simulink model "FRNmodel_IMHRC"  (Simulink 7.9)
settings: Solver=VariableStepDiscrete  StartTime=0.0  StopTime=100.0  RelTol=1e-3
libraries: simeventslib x30
(part 2 of 3)

== system FRNmodel_IMHRC/FastCartonSTORE/Calculate_INFlow ==
  Calculate_INFlow : MATLAB Function  TreatAsAtomicUnit=on
  Entity Combiner : EntityCombiner  NumberInputPorts=2
  Entity Sink : EntitySink
  Entity Splitter : EntitySplitter  NumberOutputPorts=2
  FIFO Queue : FIFOQueue  Capacity=inf
  Get Attribute : GetAttribute  AttributeName=UoH|Quantity|INFlow  AttributeMissing=Error|Error|Error  AttributeDefaultValue=1|1|1  AttributeTreatAsVector=1|1|1  AttributeSendTiming=After entity departure|After entity departure|After entity departure  EvaluatedDefaultAttributeValue={[];[];[]}
      settings: OutputPortMap=o1,o2,o3
  Set Attribute : SetAttribute  AttributeName=INFlow  AttributeFrom=Signal port  EvaluatedAttributeValue={[]}
  Single Server : SingleServer  ServiceTime=0
  FlowRecord_IN : PMIOPort  Port=1  Side=Right
  FlowRecord_OUT : PMIOPort  Port=2  Side=Right
  INFlow_Signal : PMIOPort  Port=3  Side=Left
  wires:
  Get Attribute/1 -> Calculate_INFlow/1(UoH)
  Calculate_INFlow/1(INFlow_return) -> Set Attribute/1
  Get Attribute/2 -> Calculate_INFlow/2(Quantity)
  Get Attribute/3 -> Calculate_INFlow/3(INFlow)
  connections:
  Entity Combiner/RConn1 -- Get Attribute/LConn1
  Set Attribute/RConn1 -- Entity Splitter/LConn1
  Get Attribute/RConn1 -- Single Server/LConn1
  Single Server/RConn1 -- Set Attribute/LConn1
  FlowRecord_OUT/RConn1 -- Entity Splitter/RConn1
  FlowRecord_IN/RConn1 -- Entity Combiner/LConn1
  Entity Splitter/RConn2 -- Entity Sink/LConn1
  INFlow_Signal/RConn1 -- FIFO Queue/LConn1
  FIFO Queue/RConn1 -- Entity Combiner/LConn2

== system FRNmodel_IMHRC/FastCartonSTORE/Calculate_OUTFlow ==
  Calculate_OUTFlow : MATLAB Function  TreatAsAtomicUnit=on
  Entity Combiner : EntityCombiner  NumberInputPorts=2
  Entity Sink : EntitySink
  Entity Splitter : EntitySplitter  NumberOutputPorts=2
  FIFO Queue : FIFOQueue  Capacity=inf
  Get Attribute : GetAttribute  AttributeName=UoH|Quantity|OUTFlow  AttributeMissing=Error|Error|Error  AttributeDefaultValue=1|1|1  AttributeTreatAsVector=1|1|1  AttributeSendTiming=After entity departure|After entity departure|After entity departure  EvaluatedDefaultAttributeValue={[];[];[]}
      settings: OutputPortMap=o1,o2,o3
  Set Attribute : SetAttribute  AttributeName=OUTFlow  AttributeFrom=Signal port  EvaluatedAttributeValue={[]}
  Single Server : SingleServer  ServiceTime=0
  FlowRecord_IN : PMIOPort  Port=1  Side=Left
  FlowRecord_OUT : PMIOPort  Port=2  Side=Left
  OUTFlow_Signal : PMIOPort  Port=3  Side=Right
  wires:
  Get Attribute/1 -> Calculate_OUTFlow/1(UoH)
  Calculate_OUTFlow/1(OUTFlow_return) -> Set Attribute/1
  Get Attribute/2 -> Calculate_OUTFlow/2(Quantity)
  Get Attribute/3 -> Calculate_OUTFlow/3(OUTFlow)
  connections:
  Entity Combiner/RConn1 -- Get Attribute/LConn1
  Set Attribute/RConn1 -- Entity Splitter/LConn1
  Get Attribute/RConn1 -- Single Server/LConn1
  Single Server/RConn1 -- Set Attribute/LConn1
  FlowRecord_OUT/RConn1 -- Entity Splitter/RConn1
  FlowRecord_IN/RConn1 -- Entity Combiner/LConn1
  OUTFlow_Signal/RConn1 -- FIFO Queue/LConn1
  FIFO Queue/RConn1 -- Entity Combiner/LConn2
  Entity Splitter/RConn2 -- Entity Sink/LConn1

== system FRNmodel_IMHRC/FastCartonSTORE/FRN_Process ==
  FIFO Queue1 : FIFOQueue
  N-Server : NServer  NumberOfServers=inf  ServiceTime=0
  Flow_IN : PMIOPort  Port=1  Side=Left
  Message_IN : PMIOPort  Port=2  Side=Left
  Flow_OUT : PMIOPort  Port=3  Side=Right
  Message_OUT : PMIOPort  Port=4  Side=Right
  connections:
  FIFO Queue1/RConn1 -- N-Server/LConn1
  Flow_IN/RConn1 -- FIFO Queue1/LConn1
  Flow_OUT/RConn1 -- N-Server/RConn1
  Message_OUT/RConn1 -- Message_IN/RConn1

== system FRNmodel_IMHRC/FastCartonSTORE/FlowRecord ==
  Discrete Event Signal to Workspace : simeventslib/SimEvents Sinks/Discrete Event Signal to Workspace  VariableName=INFlow_Metric  SaveFormat=Structure With Time  isMonitorOnly=off  isRecordIC=off
  Discrete Event Signal to Workspace1 : simeventslib/SimEvents Sinks/Discrete Event Signal to Workspace  VariableName=OUTFlow_Metric  SaveFormat=Structure With Time  isMonitorOnly=off  isRecordIC=off
  FIFO Queue : FIFOQueue
  FlowRecord : TimeBasedFunctionCallGenerator  EventGenerationMode=Only at simulation start
  Get Attribute : GetAttribute  AttributeName=OUTFlow|INFlow  AttributeMissing=Error|Error  AttributeDefaultValue=1|1  AttributeTreatAsVector=1|1  AttributeSendTiming=After entity departure|After entity departure  EvaluatedDefaultAttributeValue={[];[]}
      settings: OutputPortMap=o1,o2
  Initialize_FlowRecord : SetAttribute  AttributeName=INFlow|OUTFlow  AttributeFrom=Dialog|Dialog  AttributeValue=[0 0 0 0 0]|[0 0 0 0 0]  AttributeTreatAsVector=1|1  EvaluatedAttributeValue={[0 0 0 0 0];[0 0 0 0 0]}
  New_FlowRecord : EventBasedEntityGenerator  GenerateEntitiesUpon=Function call from port fcn
  Output Switch : OutputSwitch  NumberOutputPorts=2
  Path Combiner1 : PathCombiner
  TO_INFlow : PMIOPort  Port=1  Side=Right
  TO_OUTFlow : PMIOPort  Port=2  Side=Left
  FROM_INFlow : PMIOPort  Port=3  Side=Right
  FROM_OUTFlow : PMIOPort  Port=4  Side=Left
  wires:
  FlowRecord/1 -> New_FlowRecord/1
  Get Attribute/2 -> Discrete Event Signal to Workspace/1
  Get Attribute/1 -> Discrete Event Signal to Workspace1/1
  connections:
  Output Switch/LConn1 -- FIFO Queue/RConn1
  New_FlowRecord/RConn1 -- Initialize_FlowRecord/LConn1
  Initialize_FlowRecord/RConn1 -- Path Combiner1/LConn1
  TO_INFlow/RConn1 -- Output Switch/RConn1
  TO_OUTFlow/RConn1 -- Output Switch/RConn2
  FROM_INFlow/RConn1 -- Path Combiner1/LConn2
  FROM_OUTFlow/RConn1 -- Path Combiner1/LConn3
  Path Combiner1/RConn1 -- Get Attribute/LConn1
  Get Attribute/RConn1 -- FIFO Queue/LConn1

== system FRNmodel_IMHRC/HeavyCarton2MPassembly/Calculate_INFlow ==
  Calculate_INFlow : MATLAB Function  TreatAsAtomicUnit=on
  Entity Combiner : EntityCombiner  NumberInputPorts=2
  Entity Sink : EntitySink
  Entity Splitter : EntitySplitter  NumberOutputPorts=2
  FIFO Queue : FIFOQueue  Capacity=inf
  Get Attribute : GetAttribute  AttributeName=UoH|Quantity|INFlow  AttributeMissing=Error|Error|Error  AttributeDefaultValue=1|1|1  AttributeTreatAsVector=1|1|1  AttributeSendTiming=After entity departure|After entity departure|After entity departure  EvaluatedDefaultAttributeValue={[];[];[]}
      settings: OutputPortMap=o1,o2,o3
  Set Attribute : SetAttribute  AttributeName=INFlow  AttributeFrom=Signal port  EvaluatedAttributeValue={[]}
  Single Server : SingleServer  ServiceTime=0
  FlowRecord_IN : PMIOPort  Port=1  Side=Right
  FlowRecord_OUT : PMIOPort  Port=2  Side=Right
  INFlow_Signal : PMIOPort  Port=3  Side=Left
  wires:
  Get Attribute/1 -> Calculate_INFlow/1(UoH)
  Calculate_INFlow/1(INFlow_return) -> Set Attribute/1
  Get Attribute/2 -> Calculate_INFlow/2(Quantity)
  Get Attribute/3 -> Calculate_INFlow/3(INFlow)
  connections:
  Entity Combiner/RConn1 -- Get Attribute/LConn1
  Set Attribute/RConn1 -- Entity Splitter/LConn1
  Get Attribute/RConn1 -- Single Server/LConn1
  Single Server/RConn1 -- Set Attribute/LConn1
  FlowRecord_OUT/RConn1 -- Entity Splitter/RConn1
  FlowRecord_IN/RConn1 -- Entity Combiner/LConn1
  Entity Splitter/RConn2 -- Entity Sink/LConn1
  INFlow_Signal/RConn1 -- FIFO Queue/LConn1
  FIFO Queue/RConn1 -- Entity Combiner/LConn2

== system FRNmodel_IMHRC/HeavyCarton2MPassembly/Calculate_OUTFlow ==
  Calculate_OUTFlow : MATLAB Function  TreatAsAtomicUnit=on
  Entity Combiner : EntityCombiner  NumberInputPorts=2
  Entity Sink : EntitySink
  Entity Splitter : EntitySplitter  NumberOutputPorts=2
  FIFO Queue : FIFOQueue  Capacity=inf
  Get Attribute : GetAttribute  AttributeName=UoH|Quantity|OUTFlow  AttributeMissing=Error|Error|Error  AttributeDefaultValue=1|1|1  AttributeTreatAsVector=1|1|1  AttributeSendTiming=After entity departure|After entity departure|After entity departure  EvaluatedDefaultAttributeValue={[];[];[]}
      settings: OutputPortMap=o1,o2,o3
  Set Attribute : SetAttribute  AttributeName=OUTFlow  AttributeFrom=Signal port  EvaluatedAttributeValue={[]}
  Single Server : SingleServer  ServiceTime=0
  FlowRecord_IN : PMIOPort  Port=1  Side=Left
  FlowRecord_OUT : PMIOPort  Port=2  Side=Left
  OUTFlow_Signal : PMIOPort  Port=3  Side=Right
  wires:
  Get Attribute/1 -> Calculate_OUTFlow/1(UoH)
  Calculate_OUTFlow/1(OUTFlow_return) -> Set Attribute/1
  Get Attribute/2 -> Calculate_OUTFlow/2(Quantity)
  Get Attribute/3 -> Calculate_OUTFlow/3(OUTFlow)
  connections:
  Entity Combiner/RConn1 -- Get Attribute/LConn1
  Set Attribute/RConn1 -- Entity Splitter/LConn1
  Get Attribute/RConn1 -- Single Server/LConn1
  Single Server/RConn1 -- Set Attribute/LConn1
  FlowRecord_OUT/RConn1 -- Entity Splitter/RConn1
  FlowRecord_IN/RConn1 -- Entity Combiner/LConn1
  OUTFlow_Signal/RConn1 -- FIFO Queue/LConn1
  FIFO Queue/RConn1 -- Entity Combiner/LConn2
  Entity Splitter/RConn2 -- Entity Sink/LConn1

== system FRNmodel_IMHRC/HeavyCarton2MPassembly/FRN_Process ==
  FIFO Queue1 : FIFOQueue
  N-Server : NServer  NumberOfServers=inf  ServiceTime=0
  Flow_IN : PMIOPort  Port=1  Side=Left
  Message_IN : PMIOPort  Port=2  Side=Left
  Flow_OUT : PMIOPort  Port=3  Side=Right
  Message_OUT : PMIOPort  Port=4  Side=Right
  connections:
  FIFO Queue1/RConn1 -- N-Server/LConn1
  Flow_IN/RConn1 -- FIFO Queue1/LConn1
  Flow_OUT/RConn1 -- N-Server/RConn1
  Message_OUT/RConn1 -- Message_IN/RConn1

== system FRNmodel_IMHRC/HeavyCarton2MPassembly/FlowRecord ==
  Discrete Event Signal to Workspace : simeventslib/SimEvents Sinks/Discrete Event Signal to Workspace  VariableName=INFlow_Metric  SaveFormat=Structure With Time  isMonitorOnly=off  isRecordIC=off
  Discrete Event Signal to Workspace1 : simeventslib/SimEvents Sinks/Discrete Event Signal to Workspace  VariableName=OUTFlow_Metric  SaveFormat=Structure With Time  isMonitorOnly=off  isRecordIC=off
  FIFO Queue : FIFOQueue
  FlowRecord : TimeBasedFunctionCallGenerator  EventGenerationMode=Only at simulation start
  Get Attribute : GetAttribute  AttributeName=OUTFlow|INFlow  AttributeMissing=Error|Error  AttributeDefaultValue=1|1  AttributeTreatAsVector=1|1  AttributeSendTiming=After entity departure|After entity departure  EvaluatedDefaultAttributeValue={[];[]}
      settings: OutputPortMap=o1,o2
  Initialize_FlowRecord : SetAttribute  AttributeName=INFlow|OUTFlow  AttributeFrom=Dialog|Dialog  AttributeValue=[0 0 0 0 0]|[0 0 0 0 0]  AttributeTreatAsVector=1|1  EvaluatedAttributeValue={[0 0 0 0 0];[0 0 0 0 0]}
  New_FlowRecord : EventBasedEntityGenerator  GenerateEntitiesUpon=Function call from port fcn
  Output Switch : OutputSwitch  NumberOutputPorts=2
  Path Combiner1 : PathCombiner
  TO_INFlow : PMIOPort  Port=1  Side=Right
  TO_OUTFlow : PMIOPort  Port=2  Side=Left
  FROM_INFlow : PMIOPort  Port=3  Side=Right
  FROM_OUTFlow : PMIOPort  Port=4  Side=Left
  wires:
  FlowRecord/1 -> New_FlowRecord/1
  Get Attribute/2 -> Discrete Event Signal to Workspace/1
  Get Attribute/1 -> Discrete Event Signal to Workspace1/1
  connections:
  Output Switch/LConn1 -- FIFO Queue/RConn1
  New_FlowRecord/RConn1 -- Initialize_FlowRecord/LConn1
  Initialize_FlowRecord/RConn1 -- Path Combiner1/LConn1
  TO_INFlow/RConn1 -- Output Switch/RConn1
  TO_OUTFlow/RConn1 -- Output Switch/RConn2
  FROM_INFlow/RConn1 -- Path Combiner1/LConn2
  FROM_OUTFlow/RConn1 -- Path Combiner1/LConn3
  Path Combiner1/RConn1 -- Get Attribute/LConn1
  Get Attribute/RConn1 -- FIFO Queue/LConn1

== system FRNmodel_IMHRC/HeavyCartonSTORE/Calculate_INFlow ==
  Calculate_INFlow : MATLAB Function  TreatAsAtomicUnit=on
  Entity Combiner : EntityCombiner  NumberInputPorts=2
  Entity Sink : EntitySink
  Entity Splitter : EntitySplitter  NumberOutputPorts=2
  FIFO Queue : FIFOQueue  Capacity=inf
  Get Attribute : GetAttribute  AttributeName=UoH|Quantity|INFlow  AttributeMissing=Error|Error|Error  AttributeDefaultValue=1|1|1  AttributeTreatAsVector=1|1|1  AttributeSendTiming=After entity departure|After entity departure|After entity departure  EvaluatedDefaultAttributeValue={[];[];[]}
      settings: OutputPortMap=o1,o2,o3
  Set Attribute : SetAttribute  AttributeName=INFlow  AttributeFrom=Signal port  EvaluatedAttributeValue={[]}
  Single Server : SingleServer  ServiceTime=0
  FlowRecord_IN : PMIOPort  Port=1  Side=Right
  FlowRecord_OUT : PMIOPort  Port=2  Side=Right
  INFlow_Signal : PMIOPort  Port=3  Side=Left
  wires:
  Get Attribute/1 -> Calculate_INFlow/1(UoH)
  Calculate_INFlow/1(INFlow_return) -> Set Attribute/1
  Get Attribute/2 -> Calculate_INFlow/2(Quantity)
  Get Attribute/3 -> Calculate_INFlow/3(INFlow)
  connections:
  Entity Combiner/RConn1 -- Get Attribute/LConn1
  Set Attribute/RConn1 -- Entity Splitter/LConn1
  Get Attribute/RConn1 -- Single Server/LConn1
  Single Server/RConn1 -- Set Attribute/LConn1
  FlowRecord_OUT/RConn1 -- Entity Splitter/RConn1
  FlowRecord_IN/RConn1 -- Entity Combiner/LConn1
  Entity Splitter/RConn2 -- Entity Sink/LConn1
  INFlow_Signal/RConn1 -- FIFO Queue/LConn1
  FIFO Queue/RConn1 -- Entity Combiner/LConn2

== system FRNmodel_IMHRC/HeavyCartonSTORE/Calculate_OUTFlow ==
  Calculate_OUTFlow : MATLAB Function  TreatAsAtomicUnit=on
  Entity Combiner : EntityCombiner  NumberInputPorts=2
  Entity Sink : EntitySink
  Entity Splitter : EntitySplitter  NumberOutputPorts=2
  FIFO Queue : FIFOQueue  Capacity=inf
  Get Attribute : GetAttribute  AttributeName=UoH|Quantity|OUTFlow  AttributeMissing=Error|Error|Error  AttributeDefaultValue=1|1|1  AttributeTreatAsVector=1|1|1  AttributeSendTiming=After entity departure|After entity departure|After entity departure  EvaluatedDefaultAttributeValue={[];[];[]}
      settings: OutputPortMap=o1,o2,o3
  Set Attribute : SetAttribute  AttributeName=OUTFlow  AttributeFrom=Signal port  EvaluatedAttributeValue={[]}
  Single Server : SingleServer  ServiceTime=0
  FlowRecord_IN : PMIOPort  Port=1  Side=Left
  FlowRecord_OUT : PMIOPort  Port=2  Side=Left
  OUTFlow_Signal : PMIOPort  Port=3  Side=Right
  wires:
  Get Attribute/1 -> Calculate_OUTFlow/1(UoH)
  Calculate_OUTFlow/1(OUTFlow_return) -> Set Attribute/1
  Get Attribute/2 -> Calculate_OUTFlow/2(Quantity)
  Get Attribute/3 -> Calculate_OUTFlow/3(OUTFlow)
  connections:
  Entity Combiner/RConn1 -- Get Attribute/LConn1
  Set Attribute/RConn1 -- Entity Splitter/LConn1
  Get Attribute/RConn1 -- Single Server/LConn1
  Single Server/RConn1 -- Set Attribute/LConn1
  FlowRecord_OUT/RConn1 -- Entity Splitter/RConn1
  FlowRecord_IN/RConn1 -- Entity Combiner/LConn1
  OUTFlow_Signal/RConn1 -- FIFO Queue/LConn1
  FIFO Queue/RConn1 -- Entity Combiner/LConn2
  Entity Splitter/RConn2 -- Entity Sink/LConn1

== system FRNmodel_IMHRC/HeavyCartonSTORE/FRN_Process ==
  FIFO Queue1 : FIFOQueue
  N-Server : NServer  NumberOfServers=inf  ServiceTime=0
  Flow_IN : PMIOPort  Port=1  Side=Left
  Message_IN : PMIOPort  Port=2  Side=Left
  Flow_OUT : PMIOPort  Port=3  Side=Right
  Message_OUT : PMIOPort  Port=4  Side=Right
  connections:
  FIFO Queue1/RConn1 -- N-Server/LConn1
  Flow_IN/RConn1 -- FIFO Queue1/LConn1
  Flow_OUT/RConn1 -- N-Server/RConn1
  Message_OUT/RConn1 -- Message_IN/RConn1

== system FRNmodel_IMHRC/HeavyCartonSTORE/FlowRecord ==
  Discrete Event Signal to Workspace : simeventslib/SimEvents Sinks/Discrete Event Signal to Workspace  VariableName=INFlow_Metric  SaveFormat=Structure With Time  isMonitorOnly=off  isRecordIC=off
  Discrete Event Signal to Workspace1 : simeventslib/SimEvents Sinks/Discrete Event Signal to Workspace  VariableName=OUTFlow_Metric  SaveFormat=Structure With Time  isMonitorOnly=off  isRecordIC=off
  FIFO Queue : FIFOQueue
  FlowRecord : TimeBasedFunctionCallGenerator  EventGenerationMode=Only at simulation start
  Get Attribute : GetAttribute  AttributeName=OUTFlow|INFlow  AttributeMissing=Error|Error  AttributeDefaultValue=1|1  AttributeTreatAsVector=1|1  AttributeSendTiming=After entity departure|After entity departure  EvaluatedDefaultAttributeValue={[];[]}
      settings: OutputPortMap=o1,o2
  Initialize_FlowRecord : SetAttribute  AttributeName=INFlow|OUTFlow  AttributeFrom=Dialog|Dialog  AttributeValue=[0 0 0 0 0]|[0 0 0 0 0]  AttributeTreatAsVector=1|1  EvaluatedAttributeValue={[0 0 0 0 0];[0 0 0 0 0]}
  New_FlowRecord : EventBasedEntityGenerator  GenerateEntitiesUpon=Function call from port fcn
  Output Switch : OutputSwitch  NumberOutputPorts=2
  Path Combiner1 : PathCombiner
  TO_INFlow : PMIOPort  Port=1  Side=Right
  TO_OUTFlow : PMIOPort  Port=2  Side=Left
  FROM_INFlow : PMIOPort  Port=3  Side=Right
  FROM_OUTFlow : PMIOPort  Port=4  Side=Left
  wires:
  FlowRecord/1 -> New_FlowRecord/1
  Get Attribute/2 -> Discrete Event Signal to Workspace/1
  Get Attribute/1 -> Discrete Event Signal to Workspace1/1
  connections:
  Output Switch/LConn1 -- FIFO Queue/RConn1
  New_FlowRecord/RConn1 -- Initialize_FlowRecord/LConn1
  Initialize_FlowRecord/RConn1 -- Path Combiner1/LConn1
  TO_INFlow/RConn1 -- Output Switch/RConn1
  TO_OUTFlow/RConn1 -- Output Switch/RConn2
  FROM_INFlow/RConn1 -- Path Combiner1/LConn2
  FROM_OUTFlow/RConn1 -- Path Combiner1/LConn3
  Path Combiner1/RConn1 -- Get Attribute/LConn1
  Get Attribute/RConn1 -- FIFO Queue/LConn1

== system FRNmodel_IMHRC/LTL_Ship/Calculate_INFlow ==
  Calculate_INFlow : MATLAB Function  TreatAsAtomicUnit=on
  Entity Combiner : EntityCombiner  NumberInputPorts=2
  Entity Sink : EntitySink
  Entity Splitter : EntitySplitter  NumberOutputPorts=2
  FIFO Queue : FIFOQueue  Capacity=inf
  Get Attribute : GetAttribute  AttributeName=UoH|Quantity|INFlow  AttributeMissing=Error|Error|Error  AttributeDefaultValue=1|1|1  AttributeTreatAsVector=1|1|1  AttributeSendTiming=After entity departure|After entity departure|After entity departure  EvaluatedDefaultAttributeValue={[];[];[]}
      settings: OutputPortMap=o1,o2,o3
  Set Attribute : SetAttribute  AttributeName=INFlow  AttributeFrom=Signal port  EvaluatedAttributeValue={[]}
  Single Server : SingleServer  ServiceTime=0
  FlowRecord_IN : PMIOPort  Port=1  Side=Right
  FlowRecord_OUT : PMIOPort  Port=2  Side=Right
  INFlow_Signal : PMIOPort  Port=3  Side=Left
  wires:
  Get Attribute/1 -> Calculate_INFlow/1(UoH)
  Calculate_INFlow/1(INFlow_return) -> Set Attribute/1
  Get Attribute/2 -> Calculate_INFlow/2(Quantity)
  Get Attribute/3 -> Calculate_INFlow/3(INFlow)
  connections:
  Entity Combiner/RConn1 -- Get Attribute/LConn1
  Set Attribute/RConn1 -- Entity Splitter/LConn1
  Get Attribute/RConn1 -- Single Server/LConn1
  Single Server/RConn1 -- Set Attribute/LConn1
  FlowRecord_OUT/RConn1 -- Entity Splitter/RConn1
  FlowRecord_IN/RConn1 -- Entity Combiner/LConn1
  Entity Splitter/RConn2 -- Entity Sink/LConn1
  INFlow_Signal/RConn1 -- FIFO Queue/LConn1
  FIFO Queue/RConn1 -- Entity Combiner/LConn2

== system FRNmodel_IMHRC/LTL_Ship/Calculate_OUTFlow ==
  Calculate_OUTFlow : MATLAB Function  TreatAsAtomicUnit=on
  Entity Combiner : EntityCombiner  NumberInputPorts=2
  Entity Sink : EntitySink
  Entity Splitter : EntitySplitter  NumberOutputPorts=2
  FIFO Queue : FIFOQueue  Capacity=inf
  Get Attribute : GetAttribute  AttributeName=UoH|Quantity|OUTFlow  AttributeMissing=Error|Error|Error  AttributeDefaultValue=1|1|1  AttributeTreatAsVector=1|1|1  AttributeSendTiming=After entity departure|After entity departure|After entity departure  EvaluatedDefaultAttributeValue={[];[];[]}
      settings: OutputPortMap=o1,o2,o3
  Set Attribute : SetAttribute  AttributeName=OUTFlow  AttributeFrom=Signal port  EvaluatedAttributeValue={[]}
  Single Server : SingleServer  ServiceTime=0
  FlowRecord_IN : PMIOPort  Port=1  Side=Left
  FlowRecord_OUT : PMIOPort  Port=2  Side=Left
  OUTFlow_Signal : PMIOPort  Port=3  Side=Right
  wires:
  Get Attribute/1 -> Calculate_OUTFlow/1(UoH)
  Calculate_OUTFlow/1(OUTFlow_return) -> Set Attribute/1
  Get Attribute/2 -> Calculate_OUTFlow/2(Quantity)
  Get Attribute/3 -> Calculate_OUTFlow/3(OUTFlow)
  connections:
  Entity Combiner/RConn1 -- Get Attribute/LConn1
  Set Attribute/RConn1 -- Entity Splitter/LConn1
  Get Attribute/RConn1 -- Single Server/LConn1
  Single Server/RConn1 -- Set Attribute/LConn1
  FlowRecord_OUT/RConn1 -- Entity Splitter/RConn1
  FlowRecord_IN/RConn1 -- Entity Combiner/LConn1
  OUTFlow_Signal/RConn1 -- FIFO Queue/LConn1
  FIFO Queue/RConn1 -- Entity Combiner/LConn2
  Entity Splitter/RConn2 -- Entity Sink/LConn1

== system FRNmodel_IMHRC/LTL_Ship/FRN_Process ==
  FIFO Queue1 : FIFOQueue
  N-Server : NServer  NumberOfServers=inf  ServiceTime=0
  Flow_IN : PMIOPort  Port=1  Side=Left
  Message_IN : PMIOPort  Port=2  Side=Left
  Flow_OUT : PMIOPort  Port=3  Side=Right
  Message_OUT : PMIOPort  Port=4  Side=Right
  connections:
  FIFO Queue1/RConn1 -- N-Server/LConn1
  Flow_IN/RConn1 -- FIFO Queue1/LConn1
  Flow_OUT/RConn1 -- N-Server/RConn1
  Message_OUT/RConn1 -- Message_IN/RConn1

== system FRNmodel_IMHRC/LTL_Ship/FlowRecord ==
  Discrete Event Signal to Workspace : simeventslib/SimEvents Sinks/Discrete Event Signal to Workspace  VariableName=INFlow_Metric  SaveFormat=Structure With Time  isMonitorOnly=off  isRecordIC=off
  Discrete Event Signal to Workspace1 : simeventslib/SimEvents Sinks/Discrete Event Signal to Workspace  VariableName=OUTFlow_Metric  SaveFormat=Structure With Time  isMonitorOnly=off  isRecordIC=off
  FIFO Queue : FIFOQueue
  FlowRecord : TimeBasedFunctionCallGenerator  EventGenerationMode=Only at simulation start
  Get Attribute : GetAttribute  AttributeName=OUTFlow|INFlow  AttributeMissing=Error|Error  AttributeDefaultValue=1|1  AttributeTreatAsVector=1|1  AttributeSendTiming=After entity departure|After entity departure  EvaluatedDefaultAttributeValue={[];[]}
      settings: OutputPortMap=o1,o2
  Initialize_FlowRecord : SetAttribute  AttributeName=INFlow|OUTFlow  AttributeFrom=Dialog|Dialog  AttributeValue=[0 0 0 0 0]|[0 0 0 0 0]  AttributeTreatAsVector=1|1  EvaluatedAttributeValue={[0 0 0 0 0];[0 0 0 0 0]}
  New_FlowRecord : EventBasedEntityGenerator  GenerateEntitiesUpon=Function call from port fcn
  Output Switch : OutputSwitch  NumberOutputPorts=2
  Path Combiner1 : PathCombiner
  TO_INFlow : PMIOPort  Port=1  Side=Right
  TO_OUTFlow : PMIOPort  Port=2  Side=Left
  FROM_INFlow : PMIOPort  Port=3  Side=Right
  FROM_OUTFlow : PMIOPort  Port=4  Side=Left
  wires:
  FlowRecord/1 -> New_FlowRecord/1
  Get Attribute/2 -> Discrete Event Signal to Workspace/1
  Get Attribute/1 -> Discrete Event Signal to Workspace1/1
  connections:
  Output Switch/LConn1 -- FIFO Queue/RConn1
  New_FlowRecord/RConn1 -- Initialize_FlowRecord/LConn1
  Initialize_FlowRecord/RConn1 -- Path Combiner1/LConn1
  TO_INFlow/RConn1 -- Output Switch/RConn1
  TO_OUTFlow/RConn1 -- Output Switch/RConn2
  FROM_INFlow/RConn1 -- Path Combiner1/LConn2
  FROM_OUTFlow/RConn1 -- Path Combiner1/LConn3
  Path Combiner1/RConn1 -- Get Attribute/LConn1
  Get Attribute/RConn1 -- FIFO Queue/LConn1

== system FRNmodel_IMHRC/MixedCartonassembly/Calculate_INFlow ==
  Calculate_INFlow : MATLAB Function  TreatAsAtomicUnit=on
  Entity Combiner : EntityCombiner  NumberInputPorts=2
  Entity Sink : EntitySink
  Entity Splitter : EntitySplitter  NumberOutputPorts=2
  FIFO Queue : FIFOQueue  Capacity=inf
  Get Attribute : GetAttribute  AttributeName=UoH|Quantity|INFlow  AttributeMissing=Error|Error|Error  AttributeDefaultValue=1|1|1  AttributeTreatAsVector=1|1|1  AttributeSendTiming=After entity departure|After entity departure|After entity departure  EvaluatedDefaultAttributeValue={[];[];[]}
      settings: OutputPortMap=o1,o2,o3
  Set Attribute : SetAttribute  AttributeName=INFlow  AttributeFrom=Signal port  EvaluatedAttributeValue={[]}
  Single Server : SingleServer  ServiceTime=0
  FlowRecord_IN : PMIOPort  Port=1  Side=Right
  FlowRecord_OUT : PMIOPort  Port=2  Side=Right
  INFlow_Signal : PMIOPort  Port=3  Side=Left
  wires:
  Get Attribute/1 -> Calculate_INFlow/1(UoH)
  Calculate_INFlow/1(INFlow_return) -> Set Attribute/1
  Get Attribute/2 -> Calculate_INFlow/2(Quantity)
  Get Attribute/3 -> Calculate_INFlow/3(INFlow)
  connections:
  Entity Combiner/RConn1 -- Get Attribute/LConn1
  Set Attribute/RConn1 -- Entity Splitter/LConn1
  Get Attribute/RConn1 -- Single Server/LConn1
  Single Server/RConn1 -- Set Attribute/LConn1
  FlowRecord_OUT/RConn1 -- Entity Splitter/RConn1
  FlowRecord_IN/RConn1 -- Entity Combiner/LConn1
  Entity Splitter/RConn2 -- Entity Sink/LConn1
  INFlow_Signal/RConn1 -- FIFO Queue/LConn1
  FIFO Queue/RConn1 -- Entity Combiner/LConn2

== system FRNmodel_IMHRC/MixedCartonassembly/Calculate_OUTFlow ==
  Calculate_OUTFlow : MATLAB Function  TreatAsAtomicUnit=on
  Entity Combiner : EntityCombiner  NumberInputPorts=2
  Entity Sink : EntitySink
  Entity Splitter : EntitySplitter  NumberOutputPorts=2
  FIFO Queue : FIFOQueue  Capacity=inf
  Get Attribute : GetAttribute  AttributeName=UoH|Quantity|OUTFlow  AttributeMissing=Error|Error|Error  AttributeDefaultValue=1|1|1  AttributeTreatAsVector=1|1|1  AttributeSendTiming=After entity departure|After entity departure|After entity departure  EvaluatedDefaultAttributeValue={[];[];[]}
      settings: OutputPortMap=o1,o2,o3
  Set Attribute : SetAttribute  AttributeName=OUTFlow  AttributeFrom=Signal port  EvaluatedAttributeValue={[]}
  Single Server : SingleServer  ServiceTime=0
  FlowRecord_IN : PMIOPort  Port=1  Side=Left
  FlowRecord_OUT : PMIOPort  Port=2  Side=Left
  OUTFlow_Signal : PMIOPort  Port=3  Side=Right
  wires:
  Get Attribute/1 -> Calculate_OUTFlow/1(UoH)
  Calculate_OUTFlow/1(OUTFlow_return) -> Set Attribute/1
  Get Attribute/2 -> Calculate_OUTFlow/2(Quantity)
  Get Attribute/3 -> Calculate_OUTFlow/3(OUTFlow)
  connections:
  Entity Combiner/RConn1 -- Get Attribute/LConn1
  Set Attribute/RConn1 -- Entity Splitter/LConn1
  Get Attribute/RConn1 -- Single Server/LConn1
  Single Server/RConn1 -- Set Attribute/LConn1
  FlowRecord_OUT/RConn1 -- Entity Splitter/RConn1
  FlowRecord_IN/RConn1 -- Entity Combiner/LConn1
  OUTFlow_Signal/RConn1 -- FIFO Queue/LConn1
  FIFO Queue/RConn1 -- Entity Combiner/LConn2
  Entity Splitter/RConn2 -- Entity Sink/LConn1

== system FRNmodel_IMHRC/MixedCartonassembly/FRN_Process ==
  FIFO Queue1 : FIFOQueue
  N-Server : NServer  NumberOfServers=inf  ServiceTime=0
  Flow_IN : PMIOPort  Port=1  Side=Left
  Message_IN : PMIOPort  Port=2  Side=Left
  Flow_OUT : PMIOPort  Port=3  Side=Right
  Message_OUT : PMIOPort  Port=4  Side=Right
  connections:
  FIFO Queue1/RConn1 -- N-Server/LConn1
  Flow_IN/RConn1 -- FIFO Queue1/LConn1
  Flow_OUT/RConn1 -- N-Server/RConn1
  Message_OUT/RConn1 -- Message_IN/RConn1

== system FRNmodel_IMHRC/MixedCartonassembly/FlowRecord ==
  Discrete Event Signal to Workspace : simeventslib/SimEvents Sinks/Discrete Event Signal to Workspace  VariableName=INFlow_Metric  SaveFormat=Structure With Time  isMonitorOnly=off  isRecordIC=off
  Discrete Event Signal to Workspace1 : simeventslib/SimEvents Sinks/Discrete Event Signal to Workspace  VariableName=OUTFlow_Metric  SaveFormat=Structure With Time  isMonitorOnly=off  isRecordIC=off
  FIFO Queue : FIFOQueue
  FlowRecord : TimeBasedFunctionCallGenerator  EventGenerationMode=Only at simulation start
  Get Attribute : GetAttribute  AttributeName=OUTFlow|INFlow  AttributeMissing=Error|Error  AttributeDefaultValue=1|1  AttributeTreatAsVector=1|1  AttributeSendTiming=After entity departure|After entity departure  EvaluatedDefaultAttributeValue={[];[]}
      settings: OutputPortMap=o1,o2
  Initialize_FlowRecord : SetAttribute  AttributeName=INFlow|OUTFlow  AttributeFrom=Dialog|Dialog  AttributeValue=[0 0 0 0 0]|[0 0 0 0 0]  AttributeTreatAsVector=1|1  EvaluatedAttributeValue={[0 0 0 0 0];[0 0 0 0 0]}
  New_FlowRecord : EventBasedEntityGenerator  GenerateEntitiesUpon=Function call from port fcn
  Output Switch : OutputSwitch  NumberOutputPorts=2
  Path Combiner1 : PathCombiner
  TO_INFlow : PMIOPort  Port=1  Side=Right
  TO_OUTFlow : PMIOPort  Port=2  Side=Left
  FROM_INFlow : PMIOPort  Port=3  Side=Right
  FROM_OUTFlow : PMIOPort  Port=4  Side=Left
  wires:
  FlowRecord/1 -> New_FlowRecord/1
  Get Attribute/2 -> Discrete Event Signal to Workspace/1
  Get Attribute/1 -> Discrete Event Signal to Workspace1/1
  connections:
  Output Switch/LConn1 -- FIFO Queue/RConn1
  New_FlowRecord/RConn1 -- Initialize_FlowRecord/LConn1
  Initialize_FlowRecord/RConn1 -- Path Combiner1/LConn1
  TO_INFlow/RConn1 -- Output Switch/RConn1
  TO_OUTFlow/RConn1 -- Output Switch/RConn2
  FROM_INFlow/RConn1 -- Path Combiner1/LConn2
  FROM_OUTFlow/RConn1 -- Path Combiner1/LConn3
  Path Combiner1/RConn1 -- Get Attribute/LConn1
  Get Attribute/RConn1 -- FIFO Queue/LConn1

== system FRNmodel_IMHRC/MixedPalletassembly/Calculate_INFlow ==
  Calculate_INFlow : MATLAB Function  TreatAsAtomicUnit=on
  Entity Combiner : EntityCombiner  NumberInputPorts=2
  Entity Sink : EntitySink
  Entity Splitter : EntitySplitter  NumberOutputPorts=2
  FIFO Queue : FIFOQueue  Capacity=inf
  Get Attribute : GetAttribute  AttributeName=UoH|Quantity|INFlow  AttributeMissing=Error|Error|Error  AttributeDefaultValue=1|1|1  AttributeTreatAsVector=1|1|1  AttributeSendTiming=After entity departure|After entity departure|After entity departure  EvaluatedDefaultAttributeValue={[];[];[]}
      settings: OutputPortMap=o1,o2,o3
  Set Attribute : SetAttribute  AttributeName=INFlow  AttributeFrom=Signal port  EvaluatedAttributeValue={[]}
  Single Server : SingleServer  ServiceTime=0
  FlowRecord_IN : PMIOPort  Port=1  Side=Right
  FlowRecord_OUT : PMIOPort  Port=2  Side=Right
  INFlow_Signal : PMIOPort  Port=3  Side=Left
  wires:
  Get Attribute/1 -> Calculate_INFlow/1(UoH)
  Calculate_INFlow/1(INFlow_return) -> Set Attribute/1
  Get Attribute/2 -> Calculate_INFlow/2(Quantity)
  Get Attribute/3 -> Calculate_INFlow/3(INFlow)
  connections:
  Entity Combiner/RConn1 -- Get Attribute/LConn1
  Set Attribute/RConn1 -- Entity Splitter/LConn1
  Get Attribute/RConn1 -- Single Server/LConn1
  Single Server/RConn1 -- Set Attribute/LConn1
  FlowRecord_OUT/RConn1 -- Entity Splitter/RConn1
  FlowRecord_IN/RConn1 -- Entity Combiner/LConn1
  Entity Splitter/RConn2 -- Entity Sink/LConn1
  INFlow_Signal/RConn1 -- FIFO Queue/LConn1
  FIFO Queue/RConn1 -- Entity Combiner/LConn2

== system FRNmodel_IMHRC/MixedPalletassembly/Calculate_OUTFlow ==
  Calculate_OUTFlow : MATLAB Function  TreatAsAtomicUnit=on
  Entity Combiner : EntityCombiner  NumberInputPorts=2
  Entity Sink : EntitySink
  Entity Splitter : EntitySplitter  NumberOutputPorts=2
  FIFO Queue : FIFOQueue  Capacity=inf
  Get Attribute : GetAttribute  AttributeName=UoH|Quantity|OUTFlow  AttributeMissing=Error|Error|Error  AttributeDefaultValue=1|1|1  AttributeTreatAsVector=1|1|1  AttributeSendTiming=After entity departure|After entity departure|After entity departure  EvaluatedDefaultAttributeValue={[];[];[]}
      settings: OutputPortMap=o1,o2,o3
  Set Attribute : SetAttribute  AttributeName=OUTFlow  AttributeFrom=Signal port  EvaluatedAttributeValue={[]}
  Single Server : SingleServer  ServiceTime=0
  FlowRecord_IN : PMIOPort  Port=1  Side=Left
  FlowRecord_OUT : PMIOPort  Port=2  Side=Left
  OUTFlow_Signal : PMIOPort  Port=3  Side=Right
  wires:
  Get Attribute/1 -> Calculate_OUTFlow/1(UoH)
  Calculate_OUTFlow/1(OUTFlow_return) -> Set Attribute/1
  Get Attribute/2 -> Calculate_OUTFlow/2(Quantity)
  Get Attribute/3 -> Calculate_OUTFlow/3(OUTFlow)
  connections:
  Entity Combiner/RConn1 -- Get Attribute/LConn1
  Set Attribute/RConn1 -- Entity Splitter/LConn1
  Get Attribute/RConn1 -- Single Server/LConn1
  Single Server/RConn1 -- Set Attribute/LConn1
  FlowRecord_OUT/RConn1 -- Entity Splitter/RConn1
  FlowRecord_IN/RConn1 -- Entity Combiner/LConn1
  OUTFlow_Signal/RConn1 -- FIFO Queue/LConn1
  FIFO Queue/RConn1 -- Entity Combiner/LConn2
  Entity Splitter/RConn2 -- Entity Sink/LConn1

== system FRNmodel_IMHRC/MixedPalletassembly/FRN_Process ==
  FIFO Queue1 : FIFOQueue
  N-Server : NServer  NumberOfServers=inf  ServiceTime=0
  Flow_IN : PMIOPort  Port=1  Side=Left
  Message_IN : PMIOPort  Port=2  Side=Left
  Flow_OUT : PMIOPort  Port=3  Side=Right
  Message_OUT : PMIOPort  Port=4  Side=Right
  connections:
  FIFO Queue1/RConn1 -- N-Server/LConn1
  Flow_IN/RConn1 -- FIFO Queue1/LConn1
  Flow_OUT/RConn1 -- N-Server/RConn1
  Message_OUT/RConn1 -- Message_IN/RConn1

== system FRNmodel_IMHRC/MixedPalletassembly/FlowRecord ==
  Discrete Event Signal to Workspace : simeventslib/SimEvents Sinks/Discrete Event Signal to Workspace  VariableName=INFlow_Metric  SaveFormat=Structure With Time  isMonitorOnly=off  isRecordIC=off
  Discrete Event Signal to Workspace1 : simeventslib/SimEvents Sinks/Discrete Event Signal to Workspace  VariableName=OUTFlow_Metric  SaveFormat=Structure With Time  isMonitorOnly=off  isRecordIC=off
  FIFO Queue : FIFOQueue
  FlowRecord : TimeBasedFunctionCallGenerator  EventGenerationMode=Only at simulation start
  Get Attribute : GetAttribute  AttributeName=OUTFlow|INFlow  AttributeMissing=Error|Error  AttributeDefaultValue=1|1  AttributeTreatAsVector=1|1  AttributeSendTiming=After entity departure|After entity departure  EvaluatedDefaultAttributeValue={[];[]}
      settings: OutputPortMap=o1,o2
  Initialize_FlowRecord : SetAttribute  AttributeName=INFlow|OUTFlow  AttributeFrom=Dialog|Dialog  AttributeValue=[0 0 0 0 0]|[0 0 0 0 0]  AttributeTreatAsVector=1|1  EvaluatedAttributeValue={[0 0 0 0 0];[0 0 0 0 0]}
  New_FlowRecord : EventBasedEntityGenerator  GenerateEntitiesUpon=Function call from port fcn
  Output Switch : OutputSwitch  NumberOutputPorts=2
  Path Combiner1 : PathCombiner
  TO_INFlow : PMIOPort  Port=1  Side=Right
  TO_OUTFlow : PMIOPort  Port=2  Side=Left
  FROM_INFlow : PMIOPort  Port=3  Side=Right
  FROM_OUTFlow : PMIOPort  Port=4  Side=Left
  wires:
  FlowRecord/1 -> New_FlowRecord/1
  Get Attribute/2 -> Discrete Event Signal to Workspace/1
  Get Attribute/1 -> Discrete Event Signal to Workspace1/1
  connections:
  Output Switch/LConn1 -- FIFO Queue/RConn1
  New_FlowRecord/RConn1 -- Initialize_FlowRecord/LConn1
  Initialize_FlowRecord/RConn1 -- Path Combiner1/LConn1
  TO_INFlow/RConn1 -- Output Switch/RConn1
  TO_OUTFlow/RConn1 -- Output Switch/RConn2
  FROM_INFlow/RConn1 -- Path Combiner1/LConn2
  FROM_OUTFlow/RConn1 -- Path Combiner1/LConn3
  Path Combiner1/RConn1 -- Get Attribute/LConn1
  Get Attribute/RConn1 -- FIFO Queue/LConn1

== system FRNmodel_IMHRC/PickFastCarton/Calculate_INFlow ==
  Calculate_INFlow : MATLAB Function  TreatAsAtomicUnit=on
  Entity Combiner : EntityCombiner  NumberInputPorts=2
  Entity Sink : EntitySink
  Entity Splitter : EntitySplitter  NumberOutputPorts=2
  FIFO Queue : FIFOQueue  Capacity=inf
  Get Attribute : GetAttribute  AttributeName=UoH|Quantity|INFlow  AttributeMissing=Error|Error|Error  AttributeDefaultValue=1|1|1  AttributeTreatAsVector=1|1|1  AttributeSendTiming=After entity departure|After entity departure|After entity departure  EvaluatedDefaultAttributeValue={[];[];[]}
      settings: OutputPortMap=o1,o2,o3
  Set Attribute : SetAttribute  AttributeName=INFlow  AttributeFrom=Signal port  EvaluatedAttributeValue={[]}
  Single Server : SingleServer  ServiceTime=0
  FlowRecord_IN : PMIOPort  Port=1  Side=Right
  FlowRecord_OUT : PMIOPort  Port=2  Side=Right
  INFlow_Signal : PMIOPort  Port=3  Side=Left
  wires:
  Get Attribute/1 -> Calculate_INFlow/1(UoH)
  Calculate_INFlow/1(INFlow_return) -> Set Attribute/1
  Get Attribute/2 -> Calculate_INFlow/2(Quantity)
  Get Attribute/3 -> Calculate_INFlow/3(INFlow)
  connections:
  Entity Combiner/RConn1 -- Get Attribute/LConn1
  Set Attribute/RConn1 -- Entity Splitter/LConn1
  Get Attribute/RConn1 -- Single Server/LConn1
  Single Server/RConn1 -- Set Attribute/LConn1
  FlowRecord_OUT/RConn1 -- Entity Splitter/RConn1
  FlowRecord_IN/RConn1 -- Entity Combiner/LConn1
  Entity Splitter/RConn2 -- Entity Sink/LConn1
  INFlow_Signal/RConn1 -- FIFO Queue/LConn1
  FIFO Queue/RConn1 -- Entity Combiner/LConn2

== system FRNmodel_IMHRC/PickFastCarton/Calculate_OUTFlow ==
  Calculate_OUTFlow : MATLAB Function  TreatAsAtomicUnit=on
  Entity Combiner : EntityCombiner  NumberInputPorts=2
  Entity Sink : EntitySink
  Entity Splitter : EntitySplitter  NumberOutputPorts=2
  FIFO Queue : FIFOQueue  Capacity=inf
  Get Attribute : GetAttribute  AttributeName=UoH|Quantity|OUTFlow  AttributeMissing=Error|Error|Error  AttributeDefaultValue=1|1|1  AttributeTreatAsVector=1|1|1  AttributeSendTiming=After entity departure|After entity departure|After entity departure  EvaluatedDefaultAttributeValue={[];[];[]}
      settings: OutputPortMap=o1,o2,o3
  Set Attribute : SetAttribute  AttributeName=OUTFlow  AttributeFrom=Signal port  EvaluatedAttributeValue={[]}
  Single Server : SingleServer  ServiceTime=0
  FlowRecord_IN : PMIOPort  Port=1  Side=Left
  FlowRecord_OUT : PMIOPort  Port=2  Side=Left
  OUTFlow_Signal : PMIOPort  Port=3  Side=Right
  wires:
  Get Attribute/1 -> Calculate_OUTFlow/1(UoH)
  Calculate_OUTFlow/1(OUTFlow_return) -> Set Attribute/1
  Get Attribute/2 -> Calculate_OUTFlow/2(Quantity)
  Get Attribute/3 -> Calculate_OUTFlow/3(OUTFlow)
  connections:
  Entity Combiner/RConn1 -- Get Attribute/LConn1
  Set Attribute/RConn1 -- Entity Splitter/LConn1
  Get Attribute/RConn1 -- Single Server/LConn1
  Single Server/RConn1 -- Set Attribute/LConn1
  FlowRecord_OUT/RConn1 -- Entity Splitter/RConn1
  FlowRecord_IN/RConn1 -- Entity Combiner/LConn1
  OUTFlow_Signal/RConn1 -- FIFO Queue/LConn1
  FIFO Queue/RConn1 -- Entity Combiner/LConn2
  Entity Splitter/RConn2 -- Entity Sink/LConn1

== system FRNmodel_IMHRC/PickFastCarton/FRN_Process ==
  FIFO Queue1 : FIFOQueue
  N-Server : NServer  NumberOfServers=inf  ServiceTime=0
  Flow_IN : PMIOPort  Port=1  Side=Left
  Message_IN : PMIOPort  Port=2  Side=Left
  Flow_OUT : PMIOPort  Port=3  Side=Right
  Message_OUT : PMIOPort  Port=4  Side=Right
  connections:
  FIFO Queue1/RConn1 -- N-Server/LConn1
  Flow_IN/RConn1 -- FIFO Queue1/LConn1
  Flow_OUT/RConn1 -- N-Server/RConn1
  Message_OUT/RConn1 -- Message_IN/RConn1

== system FRNmodel_IMHRC/PickFastCarton/FlowRecord ==
  Discrete Event Signal to Workspace : simeventslib/SimEvents Sinks/Discrete Event Signal to Workspace  VariableName=INFlow_Metric  SaveFormat=Structure With Time  isMonitorOnly=off  isRecordIC=off
  Discrete Event Signal to Workspace1 : simeventslib/SimEvents Sinks/Discrete Event Signal to Workspace  VariableName=OUTFlow_Metric  SaveFormat=Structure With Time  isMonitorOnly=off  isRecordIC=off
  FIFO Queue : FIFOQueue
  FlowRecord : TimeBasedFunctionCallGenerator  EventGenerationMode=Only at simulation start
  Get Attribute : GetAttribute  AttributeName=OUTFlow|INFlow  AttributeMissing=Error|Error  AttributeDefaultValue=1|1  AttributeTreatAsVector=1|1  AttributeSendTiming=After entity departure|After entity departure  EvaluatedDefaultAttributeValue={[];[]}
      settings: OutputPortMap=o1,o2
  Initialize_FlowRecord : SetAttribute  AttributeName=INFlow|OUTFlow  AttributeFrom=Dialog|Dialog  AttributeValue=[0 0 0 0 0]|[0 0 0 0 0]  AttributeTreatAsVector=1|1  EvaluatedAttributeValue={[0 0 0 0 0];[0 0 0 0 0]}
  New_FlowRecord : EventBasedEntityGenerator  GenerateEntitiesUpon=Function call from port fcn
  Output Switch : OutputSwitch  NumberOutputPorts=2
  Path Combiner1 : PathCombiner
  TO_INFlow : PMIOPort  Port=1  Side=Right
  TO_OUTFlow : PMIOPort  Port=2  Side=Left
  FROM_INFlow : PMIOPort  Port=3  Side=Right
  FROM_OUTFlow : PMIOPort  Port=4  Side=Left
  wires:
  FlowRecord/1 -> New_FlowRecord/1
  Get Attribute/2 -> Discrete Event Signal to Workspace/1
  Get Attribute/1 -> Discrete Event Signal to Workspace1/1
  connections:
  Output Switch/LConn1 -- FIFO Queue/RConn1
  New_FlowRecord/RConn1 -- Initialize_FlowRecord/LConn1
  Initialize_FlowRecord/RConn1 -- Path Combiner1/LConn1
  TO_INFlow/RConn1 -- Output Switch/RConn1
  TO_OUTFlow/RConn1 -- Output Switch/RConn2
  FROM_INFlow/RConn1 -- Path Combiner1/LConn2
  FROM_OUTFlow/RConn1 -- Path Combiner1/LConn3
  Path Combiner1/RConn1 -- Get Attribute/LConn1
  Get Attribute/RConn1 -- FIFO Queue/LConn1

== system FRNmodel_IMHRC/PickHeavyCarton/Calculate_INFlow ==
  Calculate_INFlow : MATLAB Function  TreatAsAtomicUnit=on
  Entity Combiner : EntityCombiner  NumberInputPorts=2
  Entity Sink : EntitySink
  Entity Splitter : EntitySplitter  NumberOutputPorts=2
  FIFO Queue : FIFOQueue  Capacity=inf
  Get Attribute : GetAttribute  AttributeName=UoH|Quantity|INFlow  AttributeMissing=Error|Error|Error  AttributeDefaultValue=1|1|1  AttributeTreatAsVector=1|1|1  AttributeSendTiming=After entity departure|After entity departure|After entity departure  EvaluatedDefaultAttributeValue={[];[];[]}
      settings: OutputPortMap=o1,o2,o3
  Set Attribute : SetAttribute  AttributeName=INFlow  AttributeFrom=Signal port  EvaluatedAttributeValue={[]}
  Single Server : SingleServer  ServiceTime=0
  FlowRecord_IN : PMIOPort  Port=1  Side=Right
  FlowRecord_OUT : PMIOPort  Port=2  Side=Right
  INFlow_Signal : PMIOPort  Port=3  Side=Left
  wires:
  Get Attribute/1 -> Calculate_INFlow/1(UoH)
  Calculate_INFlow/1(INFlow_return) -> Set Attribute/1
  Get Attribute/2 -> Calculate_INFlow/2(Quantity)
  Get Attribute/3 -> Calculate_INFlow/3(INFlow)
  connections:
  Entity Combiner/RConn1 -- Get Attribute/LConn1
  Set Attribute/RConn1 -- Entity Splitter/LConn1
  Get Attribute/RConn1 -- Single Server/LConn1
  Single Server/RConn1 -- Set Attribute/LConn1
  FlowRecord_OUT/RConn1 -- Entity Splitter/RConn1
  FlowRecord_IN/RConn1 -- Entity Combiner/LConn1
  Entity Splitter/RConn2 -- Entity Sink/LConn1
  INFlow_Signal/RConn1 -- FIFO Queue/LConn1
  FIFO Queue/RConn1 -- Entity Combiner/LConn2

== system FRNmodel_IMHRC/PickHeavyCarton/Calculate_OUTFlow ==
  Calculate_OUTFlow : MATLAB Function  TreatAsAtomicUnit=on
  Entity Combiner : EntityCombiner  NumberInputPorts=2
  Entity Sink : EntitySink
  Entity Splitter : EntitySplitter  NumberOutputPorts=2
  FIFO Queue : FIFOQueue  Capacity=inf
  Get Attribute : GetAttribute  AttributeName=UoH|Quantity|OUTFlow  AttributeMissing=Error|Error|Error  AttributeDefaultValue=1|1|1  AttributeTreatAsVector=1|1|1  AttributeSendTiming=After entity departure|After entity departure|After entity departure  EvaluatedDefaultAttributeValue={[];[];[]}
      settings: OutputPortMap=o1,o2,o3
  Set Attribute : SetAttribute  AttributeName=OUTFlow  AttributeFrom=Signal port  EvaluatedAttributeValue={[]}
  Single Server : SingleServer  ServiceTime=0
  FlowRecord_IN : PMIOPort  Port=1  Side=Left
  FlowRecord_OUT : PMIOPort  Port=2  Side=Left
  OUTFlow_Signal : PMIOPort  Port=3  Side=Right
  wires:
  Get Attribute/1 -> Calculate_OUTFlow/1(UoH)
  Calculate_OUTFlow/1(OUTFlow_return) -> Set Attribute/1
  Get Attribute/2 -> Calculate_OUTFlow/2(Quantity)
  Get Attribute/3 -> Calculate_OUTFlow/3(OUTFlow)
  connections:
  Entity Combiner/RConn1 -- Get Attribute/LConn1
  Set Attribute/RConn1 -- Entity Splitter/LConn1
  Get Attribute/RConn1 -- Single Server/LConn1
  Single Server/RConn1 -- Set Attribute/LConn1
  FlowRecord_OUT/RConn1 -- Entity Splitter/RConn1
  FlowRecord_IN/RConn1 -- Entity Combiner/LConn1
  OUTFlow_Signal/RConn1 -- FIFO Queue/LConn1
  FIFO Queue/RConn1 -- Entity Combiner/LConn2
  Entity Splitter/RConn2 -- Entity Sink/LConn1

== system FRNmodel_IMHRC/PickHeavyCarton/FRN_Process ==
  FIFO Queue1 : FIFOQueue
  N-Server : NServer  NumberOfServers=inf  ServiceTime=0
  Flow_IN : PMIOPort  Port=1  Side=Left
  Message_IN : PMIOPort  Port=2  Side=Left
  Flow_OUT : PMIOPort  Port=3  Side=Right
  Message_OUT : PMIOPort  Port=4  Side=Right
  connections:
  FIFO Queue1/RConn1 -- N-Server/LConn1
  Flow_IN/RConn1 -- FIFO Queue1/LConn1
  Flow_OUT/RConn1 -- N-Server/RConn1
  Message_OUT/RConn1 -- Message_IN/RConn1

== system FRNmodel_IMHRC/PickHeavyCarton/FlowRecord ==
  Discrete Event Signal to Workspace : simeventslib/SimEvents Sinks/Discrete Event Signal to Workspace  VariableName=INFlow_Metric  SaveFormat=Structure With Time  isMonitorOnly=off  isRecordIC=off
  Discrete Event Signal to Workspace1 : simeventslib/SimEvents Sinks/Discrete Event Signal to Workspace  VariableName=OUTFlow_Metric  SaveFormat=Structure With Time  isMonitorOnly=off  isRecordIC=off
  FIFO Queue : FIFOQueue
  FlowRecord : TimeBasedFunctionCallGenerator  EventGenerationMode=Only at simulation start
  Get Attribute : GetAttribute  AttributeName=OUTFlow|INFlow  AttributeMissing=Error|Error  AttributeDefaultValue=1|1  AttributeTreatAsVector=1|1  AttributeSendTiming=After entity departure|After entity departure  EvaluatedDefaultAttributeValue={[];[]}
      settings: OutputPortMap=o1,o2
  Initialize_FlowRecord : SetAttribute  AttributeName=INFlow|OUTFlow  AttributeFrom=Dialog|Dialog  AttributeValue=[0 0 0 0 0]|[0 0 0 0 0]  AttributeTreatAsVector=1|1  EvaluatedAttributeValue={[0 0 0 0 0];[0 0 0 0 0]}
  New_FlowRecord : EventBasedEntityGenerator  GenerateEntitiesUpon=Function call from port fcn
  Output Switch : OutputSwitch  NumberOutputPorts=2
  Path Combiner1 : PathCombiner
  TO_INFlow : PMIOPort  Port=1  Side=Right
  TO_OUTFlow : PMIOPort  Port=2  Side=Left
  FROM_INFlow : PMIOPort  Port=3  Side=Right
  FROM_OUTFlow : PMIOPort  Port=4  Side=Left
  wires:
  FlowRecord/1 -> New_FlowRecord/1
  Get Attribute/2 -> Discrete Event Signal to Workspace/1
  Get Attribute/1 -> Discrete Event Signal to Workspace1/1
  connections:
  Output Switch/LConn1 -- FIFO Queue/RConn1
  New_FlowRecord/RConn1 -- Initialize_FlowRecord/LConn1
  Initialize_FlowRecord/RConn1 -- Path Combiner1/LConn1
  TO_INFlow/RConn1 -- Output Switch/RConn1
  TO_OUTFlow/RConn1 -- Output Switch/RConn2
  FROM_INFlow/RConn1 -- Path Combiner1/LConn2
  FROM_OUTFlow/RConn1 -- Path Combiner1/LConn3
  Path Combiner1/RConn1 -- Get Attribute/LConn1
  Get Attribute/RConn1 -- FIFO Queue/LConn1

== system FRNmodel_IMHRC/PickSlowCarton/Calculate_INFlow ==
  Calculate_INFlow : MATLAB Function  TreatAsAtomicUnit=on
  Entity Combiner : EntityCombiner  NumberInputPorts=2
  Entity Sink : EntitySink
  Entity Splitter : EntitySplitter  NumberOutputPorts=2
  FIFO Queue : FIFOQueue  Capacity=inf
  Get Attribute : GetAttribute  AttributeName=UoH|Quantity|INFlow  AttributeMissing=Error|Error|Error  AttributeDefaultValue=1|1|1  AttributeTreatAsVector=1|1|1  AttributeSendTiming=After entity departure|After entity departure|After entity departure  EvaluatedDefaultAttributeValue={[];[];[]}
      settings: OutputPortMap=o1,o2,o3
  Set Attribute : SetAttribute  AttributeName=INFlow  AttributeFrom=Signal port  EvaluatedAttributeValue={[]}
  Single Server : SingleServer  ServiceTime=0
  FlowRecord_IN : PMIOPort  Port=1  Side=Right
  FlowRecord_OUT : PMIOPort  Port=2  Side=Right
  INFlow_Signal : PMIOPort  Port=3  Side=Left
  wires:
  Get Attribute/1 -> Calculate_INFlow/1(UoH)
  Calculate_INFlow/1(INFlow_return) -> Set Attribute/1
  Get Attribute/2 -> Calculate_INFlow/2(Quantity)
  Get Attribute/3 -> Calculate_INFlow/3(INFlow)
  connections:
  Entity Combiner/RConn1 -- Get Attribute/LConn1
  Set Attribute/RConn1 -- Entity Splitter/LConn1
  Get Attribute/RConn1 -- Single Server/LConn1
  Single Server/RConn1 -- Set Attribute/LConn1
  FlowRecord_OUT/RConn1 -- Entity Splitter/RConn1
  FlowRecord_IN/RConn1 -- Entity Combiner/LConn1
  Entity Splitter/RConn2 -- Entity Sink/LConn1
  INFlow_Signal/RConn1 -- FIFO Queue/LConn1
  FIFO Queue/RConn1 -- Entity Combiner/LConn2

== system FRNmodel_IMHRC/PickSlowCarton/Calculate_OUTFlow ==
  Calculate_OUTFlow : MATLAB Function  TreatAsAtomicUnit=on
  Entity Combiner : EntityCombiner  NumberInputPorts=2
  Entity Sink : EntitySink
  Entity Splitter : EntitySplitter  NumberOutputPorts=2
  FIFO Queue : FIFOQueue  Capacity=inf
  Get Attribute : GetAttribute  AttributeName=UoH|Quantity|OUTFlow  AttributeMissing=Error|Error|Error  AttributeDefaultValue=1|1|1  AttributeTreatAsVector=1|1|1  AttributeSendTiming=After entity departure|After entity departure|After entity departure  EvaluatedDefaultAttributeValue={[];[];[]}
      settings: OutputPortMap=o1,o2,o3
  Set Attribute : SetAttribute  AttributeName=OUTFlow  AttributeFrom=Signal port  EvaluatedAttributeValue={[]}
  Single Server : SingleServer  ServiceTime=0
  FlowRecord_IN : PMIOPort  Port=1  Side=Left
  FlowRecord_OUT : PMIOPort  Port=2  Side=Left
  OUTFlow_Signal : PMIOPort  Port=3  Side=Right
  wires:
  Get Attribute/1 -> Calculate_OUTFlow/1(UoH)
  Calculate_OUTFlow/1(OUTFlow_return) -> Set Attribute/1
  Get Attribute/2 -> Calculate_OUTFlow/2(Quantity)
  Get Attribute/3 -> Calculate_OUTFlow/3(OUTFlow)
  connections:
  Entity Combiner/RConn1 -- Get Attribute/LConn1
  Set Attribute/RConn1 -- Entity Splitter/LConn1
  Get Attribute/RConn1 -- Single Server/LConn1
  Single Server/RConn1 -- Set Attribute/LConn1
  FlowRecord_OUT/RConn1 -- Entity Splitter/RConn1
  FlowRecord_IN/RConn1 -- Entity Combiner/LConn1
  OUTFlow_Signal/RConn1 -- FIFO Queue/LConn1
  FIFO Queue/RConn1 -- Entity Combiner/LConn2
  Entity Splitter/RConn2 -- Entity Sink/LConn1

== system FRNmodel_IMHRC/PickSlowCarton/FRN_Process ==
  FIFO Queue1 : FIFOQueue
  N-Server : NServer  NumberOfServers=inf  ServiceTime=0
  Flow_IN : PMIOPort  Port=1  Side=Left
  Message_IN : PMIOPort  Port=2  Side=Left
  Flow_OUT : PMIOPort  Port=3  Side=Right
  Message_OUT : PMIOPort  Port=4  Side=Right
  connections:
  FIFO Queue1/RConn1 -- N-Server/LConn1
  Flow_IN/RConn1 -- FIFO Queue1/LConn1
  Flow_OUT/RConn1 -- N-Server/RConn1
  Message_OUT/RConn1 -- Message_IN/RConn1
